simulink model "fwv_modified"  (R2021b)
settings: Solver=ode15s  StartTime=0.0  StopTime=10  FixedStep=0.01  MaxStep=0.01  RelTol=1e-3  AbsTol=1e-3  EnableMultiTasking=on
model workspace (MATLAB code in the model file):
  | p0=[0 0 0];
undefined symbols (not defined in the file): A_D, A_L, adpk, adps, c_bar, C_D0, il, ol, psi0, r00, r11, r22, r33, r_cp, rho, Rw, X, Y, Z, z00, z11, z22, zrd
libraries: sm_lib x54, nesl_utility x45, vrlib x3
(part 3 of 3)

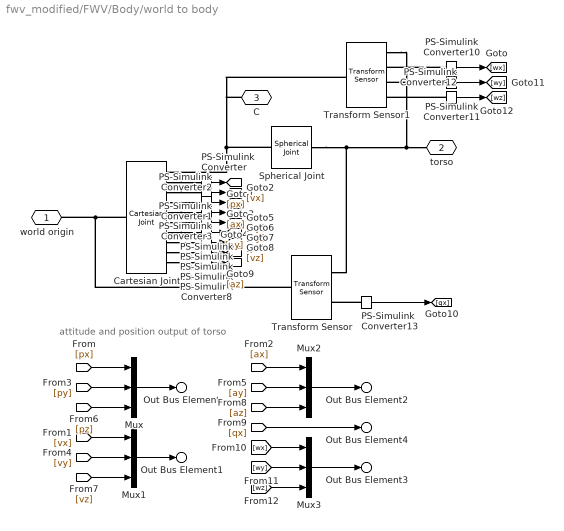
== system fwv_modified/FWV/Body/world to body ==
  note: attitude and position output of torso
  Cartesian Joint : sm_lib/Joints/Cartesian Joint  JointMode=Normal  SenseConstraintForce=off  SenseConstraintForceX=off  SenseConstraintForceY=off  SenseConstraintForceZ=off  SenseConstraintTorque=off  SenseConstraintTorqueX=off  SenseConstraintTorqueY=off  SenseConstraintTorqueZ=off  SenseTotalForce=off  SenseTotalForceX=off  SenseTotalForceY=off  SenseTotalForceZ=off  SenseTotalTorque=off  SenseTotalTorqueX=off  SenseTotalTorqueY=off  SenseTotalTorqueZ=off  CompositeWrenchDir=FollowerOnBase  CompositeWrenchFrame=BaseFrame  PxEquilibriumPosition=0  PxEquilibriumPositionUnits=m  PxSpringStiffness=0  PxSpringStiffnessUnits=N/m  PxDampingCoefficient=0  PxDampingCoefficientUnits=N/(m/s)  PxTorqueActuationMode=NoTorque  PxMotionActuationMode=ComputedMotion  PxSensePosition=on  PxSenseVelocity=on  PxSenseAcceleration=on  PxSenseTorqueForce=off  PxSenseLowerLimitTorqueForce=off  PxSenseUpperLimitTorqueForce=off  PxLowerLimitSpecify=off  PxLowerLimitBound=-1  PxLowerLimitBoundUnits=m  PxLowerLimitStiffness=1e6  PxLowerLimitStiffnessUnits=N/m  PxLowerLimitDamping=1e3  PxLowerLimitDampingUnits=N/(m/s)  PxLowerLimitTransitionRegionWidth=1e-4  PxLowerLimitTransitionRegionWidthUnits=m  PxUpperLimitSpecify=off  PxUpperLimitBound=1  PxUpperLimitBoundUnits=m  PxUpperLimitStiffness=1e6  PxUpperLimitStiffnessUnits=N/m  PxUpperLimitDamping=1e3  PxUpperLimitDampingUnits=N/(m/s)  PxUpperLimitTransitionRegionWidth=1e-4  PxUpperLimitTransitionRegionWidthUnits=m  PxPositionTargetSpecify=on  PxPositionTargetPriority=High  PxPositionTargetValue=p0(1)  PxPositionTargetValueUnits=m  PxVelocityTargetSpecify=off  PxVelocityTargetPriority=High  PxVelocityTargetValue=0  PxVelocityTargetValueUnits=m/s  PyEquilibriumPosition=0  PyEquilibriumPositionUnits=m  PySpringStiffness=0  PySpringStiffnessUnits=N/m  PyDampingCoefficient=0  PyDampingCoefficientUnits=N/(m/s)  PyTorqueActuationMode=NoTorque  PyMotionActuationMode=ComputedMotion  PySensePosition=on  PySenseVelocity=on  PySenseAcceleration=on  PySenseTorqueForce=off  PySenseLowerLimitTorqueForce=off  PySenseUpperLimitTorqueForce=off  PyLowerLimitSpecify=off  PyLowerLimitBound=-1  PyLowerLimitBoundUnits=m  PyLowerLimitStiffness=1e6  PyLowerLimitStiffnessUnits=N/m  PyLowerLimitDamping=1e3  PyLowerLimitDampingUnits=N/(m/s)  PyLowerLimitTransitionRegionWidth=1e-4  PyLowerLimitTransitionRegionWidthUnits=m  PyUpperLimitSpecify=off  PyUpperLimitBound=1  PyUpperLimitBoundUnits=m  PyUpperLimitStiffness=1e6  PyUpperLimitStiffnessUnits=N/m  PyUpperLimitDamping=1e3  PyUpperLimitDampingUnits=N/(m/s)  PyUpperLimitTransitionRegionWidth=1e-4  PyUpperLimitTransitionRegionWidthUnits=m  PyPositionTargetSpecify=on  PyPositionTargetPriority=High  PyPositionTargetValue=p0(2)  PyPositionTargetValueUnits=m  PyVelocityTargetSpecify=off  PyVelocityTargetPriority=High  PyVelocityTargetValue=0  PyVelocityTargetValueUnits=m/s  PzEquilibriumPosition=0  PzEquilibriumPositionUnits=m  PzSpringStiffness=0  PzSpringStiffnessUnits=N/m  PzDampingCoefficient=0  PzDampingCoefficientUnits=N/(m/s)  PzTorqueActuationMode=NoTorque  PzMotionActuationMode=ComputedMotion  PzSensePosition=on  PzSenseVelocity=on  PzSenseAcceleration=on  PzSenseTorqueForce=off  PzSenseLowerLimitTorqueForce=off  PzSenseUpperLimitTorqueForce=off  PzLowerLimitSpecify=off  PzLowerLimitBound=-1  PzLowerLimitBoundUnits=m  PzLowerLimitStiffness=1e6  PzLowerLimitStiffnessUnits=N/m  PzLowerLimitDamping=1e3  PzLowerLimitDampingUnits=N/(m/s)  PzLowerLimitTransitionRegionWidth=1e-4  PzLowerLimitTransitionRegionWidthUnits=m  PzUpperLimitSpecify=off  PzUpperLimitBound=1  PzUpperLimitBoundUnits=m  PzUpperLimitStiffness=1e6  PzUpperLimitStiffnessUnits=N/m  PzUpperLimitDamping=1e3  PzUpperLimitDampingUnits=N/(m/s)  PzUpperLimitTransitionRegionWidth=1e-4  PzUpperLimitTransitionRegionWidthUnits=m  PzPositionTargetSpecify=on  PzPositionTargetPriority=High  PzPositionTargetValue=p0(3)  PzPositionTargetValueUnits=m  PzVelocityTargetSpecify=off  PzVelocityTargetPriority=High  PzVelocityTargetValue=0  PzVelocityTargetValueUnits=m/s
  Mux{,1..3} (4 alike) : Mux  Inputs=3
  PS-Simulink Converter{,1..8,10..13} (13 alike) : nesl_utility/PS-Simulink Converter  PhysicalDomain=network_engine_domain  SubClassName=ps_output  LeftPortType=input  RightPortType=output  PseudoPeriodic=off  Frequencies=[]  Unit=inherit  AffineConversion=off
      settings: SourceProductBaseCode=PW,SS
  Spherical Joint : sm_lib/Joints/Spherical Joint  JointMode=Normal  SenseConstraintForce=off  SenseConstraintForceX=off  SenseConstraintForceY=off  SenseConstraintForceZ=off  SenseConstraintTorque=off  SenseConstraintTorqueX=off  SenseConstraintTorqueY=off  SenseConstraintTorqueZ=off  SenseTotalForce=off  SenseTotalForceX=off  SenseTotalForceY=off  SenseTotalForceZ=off  SenseTotalTorque=off  SenseTotalTorqueX=off  SenseTotalTorqueY=off  SenseTotalTorqueZ=off  CompositeWrenchDir=FollowerOnBase  CompositeWrenchFrame=BaseFrame  DefPosRotationMethod=None  DefPosRotationAngleUnits=deg  DefPosRotationStandardAxis=+Z  DefPosRotationAngle=0.0  DefPosRotationArbitraryAxis=[0 0 1]  DefPosFollAlignAxisA=+X  DefPosBaseAlignAxisA=+Y  DefPosFollAlignAxisB=+Y  DefPosBaseAlignAxisB=+Z  DefPosRotationSequenceAxes=FollowerAxes  DefPosRotationSequence=XYX  DefPosRotationSequenceAngles=[0 0 0]  DefPosRotationSequenceAnglesUnits=deg  DefPosRotationMatrix=[1 0 0; 0 1 0; 0 0 1]  EqPosRotationMethod=None  EqPosRotationAngleUnits=deg  EqPosRotationStandardAxis=+Z  EqPosRotationAngle=0.0  EqPosRotationArbitraryAxis=[0 0 1]  EqPosFollAlignAxisA=+X  EqPosBaseAlignAxisA=+Y  EqPosFollAlignAxisB=+Y  EqPosBaseAlignAxisB=+Z  EqPosRotationSequenceAxes=FollowerAxes  EqPosRotationSequence=XYX  EqPosRotationSequenceAngles=[0 0 0]  EqPosRotationSequenceAnglesUnits=deg  EqPosRotationMatrix=[1 0 0; 0 1 0; 0 0 1]  SpringStiffness=0  SpringStiffnessUnits=N*m/deg  DampingCoefficient=0  DampingCoefficientUnits=N*m/(deg/s)  ActuateTorqueX=off  ActuateTorqueY=off  ActuateTorqueZ=off  ActuateTorque=off  TorqueActuationMode=NoTorque  MotionActuationMode=ComputedMotion  ActuationFrame=BaseFrame  SensePosition=off  SenseVelocityX=off  SenseVelocityY=off  SenseVelocityZ=off  SenseVelocity=off  SenseAccelerationX=off  SenseAccelerationY=off  SenseAccelerationZ=off  SenseAcceleration=off  SenseTorqueX=off  SenseTorqueY=off  SenseTorqueZ=off  SenseTorqueForce=off  SenseLowerLimitTorqueMag=off  SenseUpperLimitTorqueMag=off  SensingFrame=BaseFrame  LowerLimitSpecify=off  LowerLimitBound=15  LowerLimitBoundUnits=deg  LowerLimitStiffness=1e4  LowerLimitStiffnessUnits=N*m/deg  LowerLimitDamping=10  LowerLimitDampingUnits=N*m/(deg/s)  LowerLimitTransitionRegionWidth=0.1  LowerLimitTransitionRegionWidthUnits=deg  UpperLimitSpecify=off  UpperLimitBound=45  UpperLimitBoundUnits=deg  UpperLimitStiffness=1e4  UpperLimitStiffnessUnits=N*m/deg  UpperLimitDamping=10  UpperLimitDampingUnits=N*m/(deg/s)  UpperLimitTransitionRegionWidth=0.1  UpperLimitTransitionRegionWidthUnits=deg  PositionTargetRotationMethod=RotationSequence  PositionTargetRotationAngleUnits=deg  PositionTargetRotationStandardAxis=+Z  PositionTargetRotationAngle=0.0  PositionTargetRotationArbitraryAxis=[0 0 1]  PositionTargetFollAlignAxisA=+X  PositionTargetBaseAlignAxisA=+Y  PositionTargetFollAlignAxisB=+Y  PositionTargetBaseAlignAxisB=+Z  PositionTargetRotationSequenceAxes=FollowerAxes  PositionTargetRotationSequence=ZYX  PositionTargetRotationSequenceAngles=[psi0 theta0 phi0]  PositionTargetRotationSequenceAnglesUnits=rad  PositionTargetRotationMatrix=[1 0 0; 0 1 0; 0 0 1]  PositionTargetSpecify=on  PositionTargetPriority=High  VelocityTargetValue=[0 0 0]  VelocityTargetValueUnits=deg/s  VelocityTargetSpecify=off  VelocityTargetPriority=High  VelocityTargetInFollowerFrame=on
  Transform Sensor : sm_lib/Frames and Transforms/Transform Sensor  MeasurementFrame=NonRotatingBase  SenseAngle=off  SenseAxis=off  SenseAngle1=off  SenseAngle2=off  SenseAngle3=off  SenseQ=off  SenseR=on  SenseOmegaX=off  SenseOmegaY=off  SenseOmegaZ=off  SenseOmega1=off  SenseOmega2=off  SenseOmega3=off  SenseQDot=off  SenseRDot=off  SenseAlphaX=off  SenseAlphaY=off  SenseAlphaZ=off  SenseAlpha1=off  SenseAlpha2=off  SenseAlpha3=off  SenseQDDot=off  SenseRDDot=off  SenseX=off  SenseY=off  SenseZ=off  SenseRad=off  SenseAzim=off  SenseDist=off  SenseInc=off  SenseXDot=off  SenseYDot=off  SenseZDot=off  SenseRadDot=off  SenseAzimDot=off  SenseDistDot=off  SenseIncDot=off  SenseXDDot=off  SenseYDDot=off  SenseZDDot=off  SenseRadDDot=off  SenseAzimDDot=off  SenseDistDDot=off  SenseIncDDot=off
  Transform Sensor1 : sm_lib/Frames and Transforms/Transform Sensor  MeasurementFrame=NonRotatingFollower  SenseAngle=off  SenseAxis=off  SenseAngle1=off  SenseAngle2=off  SenseAngle3=off  SenseQ=off  SenseR=off  SenseOmegaX=on  SenseOmegaY=on  SenseOmegaZ=on  SenseOmega1=off  SenseOmega2=off  SenseOmega3=off  SenseQDot=off  SenseRDot=off  SenseAlphaX=off  SenseAlphaY=off  SenseAlphaZ=off  SenseAlpha1=off  SenseAlpha2=off  SenseAlpha3=off  SenseQDDot=off  SenseRDDot=off  SenseX=off  SenseY=off  SenseZ=off  SenseRad=off  SenseAzim=off  SenseDist=off  SenseInc=off  SenseXDot=off  SenseYDot=off  SenseZDot=off  SenseRadDot=off  SenseAzimDot=off  SenseDistDot=off  SenseIncDot=off  SenseXDDot=off  SenseYDDot=off  SenseZDDot=off  SenseRadDDot=off  SenseAzimDDot=off  SenseDistDDot=off  SenseIncDDot=off
  world origin : PMIOPort  Side=Left
  torso : PMIOPort  Port=2  Side=Right
  C : PMIOPort  Port=3  Side=Left
  Out Bus Element : Outport  PortName=torso_  Element=p
  Out Bus Element1 : Outport  PortName=torso_  Element=v
  Out Bus Element2 : Outport  PortName=torso_  Element=a
  Out Bus Element3 : Outport  PortName=torso_  Element=w
  Out Bus Element4 : Outport  PortName=torso_  Element=R
  wires:
  [vy] -> Mux1/2
  [px] -> Mux/1
  [ax] -> Mux2/1
  [vz] -> Mux1/3
  Mux1/1 -> Out Bus Element1/1
  [az] -> Mux2/3
  [vx] -> Mux1/1
  [ay] -> Mux2/2
  [pz] -> Mux/3
  Mux/1 -> Out Bus Element/1
  Mux2/1 -> Out Bus Element2/1
  [py] -> Mux/2
  PS-Simulink Converter7/1 -> [vz]
  PS-Simulink Converter4/1 -> [vy]
  PS-Simulink Converter5/1 -> [ay]
  PS-Simulink Converter1/1 -> [vx]
  PS-Simulink Converter3/1 -> [py]
  PS-Simulink Converter/1 -> [px]
  PS-Simulink Converter2/1 -> [ax]
  PS-Simulink Converter6/1 -> [pz]
  PS-Simulink Converter8/1 -> [az]
  [qx] -> Out Bus Element4/1
  PS-Simulink Converter13/1 -> [qx]
  PS-Simulink Converter10/1 -> [wx]
  PS-Simulink Converter11/1 -> [wy]
  PS-Simulink Converter12/1 -> [wz]
  Mux3/1 -> Out Bus Element3/1
  [wx] -> Mux3/1
  [wy] -> Mux3/2
  [wz] -> Mux3/3
  connections:
  Cartesian Joint/LConn1 -- world origin/RConn1 -- Transform Sensor/LConn1
  Transform Sensor/RConn1 -- Transform Sensor1/RConn1 -- torso/RConn1 -- Spherical Joint/RConn1
  Spherical Joint/LConn1 -- Transform Sensor1/LConn1 -- C/RConn1 -- Cartesian Joint/RConn1
  PS-Simulink Converter13/LConn1 -- Transform Sensor/RConn2
  Cartesian Joint/RConn2 -- PS-Simulink Converter/LConn1
  Cartesian Joint/RConn3 -- PS-Simulink Converter1/LConn1
  Cartesian Joint/RConn4 -- PS-Simulink Converter2/LConn1
  Cartesian Joint/RConn5 -- PS-Simulink Converter3/LConn1
  Cartesian Joint/RConn6 -- PS-Simulink Converter4/LConn1
  Cartesian Joint/RConn7 -- PS-Simulink Converter5/LConn1
  Cartesian Joint/RConn8 -- PS-Simulink Converter6/LConn1
  Cartesian Joint/RConn9 -- PS-Simulink Converter7/LConn1
  Cartesian Joint/RConn10 -- PS-Simulink Converter8/LConn1
  PS-Simulink Converter10/LConn1 -- Transform Sensor1/RConn2
  PS-Simulink Converter11/LConn1 -- Transform Sensor1/RConn3
  PS-Simulink Converter12/LConn1 -- Transform Sensor1/RConn4

== system fwv_modified/FWV/Controller/Inner PD ==
  eR : Inport
  omega : Inport  Port=2
  Add : Sum  Inputs=---
  Integrator : Integrator  Commented=on  InitialCondition=[0; 0; 0]
  Kd : Constant  Value=diag(il.Kd)
  Kp : Constant  Value=diag(il.Kp)
  Multiply : Gain  Commented=on  Gain=[0.1 0.1 0]
  Product : Product  Multiplication=Matrix(*)
  Product1 : Product  Multiplication=Matrix(*)
  Scope : Scope  NumInputPorts=2
  Selector : Selector  InputPortWidth=3  IndexOptions=Index vector (dialog)  Indices=[2]  OutputSizes=1
  Selector1 : Selector  InputPortWidth=3  IndexOptions=Index vector (dialog)  Indices=[2]  OutputSizes=1
  get P : Subsystem
  to euler1 : Subsystem
  tau_d : Outport
  wires:
  eR/1 -> to euler1/1(R), get P/1(eR)
  Kp/1 -> Product/1
  get P/1(Out) -> Integrator/1, Product/2
  Add/1 -> tau_d/1
  Product1/1 -> Selector1/1, Add/3
  Kd/1 -> Product1/1
  Product/1 -> Selector/1, Add/1
  Selector/1 -> Scope/1
  Selector1/1 -> Scope/2
  omega/1 -> Product1/2
  Integrator/1 -> Multiply/1
  Multiply/1 -> Add/2

== system fwv_modified/FWV/Controller/Mean3 ==
  In1 : Inport
  Add : Sum  Inputs=+-
  Gain : Gain  Gain=1/0.04
  Integrator : Integrator  ZeroCross=off
  Transport Delay : TransportDelay  DelayTime=0.04  InitialOutput=p0  BufferSize=4096
  Mean1 : Outport
  wires:
  In1/1 -> Integrator/1
  Integrator/1 -> Transport Delay/1, Add/1
  Transport Delay/1 -> Add/2
  Add/1 -> Gain/1
  Gain/1 -> Mean1/1

== system fwv_modified/FWV/Controller/Mean4 ==
  In1 : Inport
  Add : Sum  Inputs=+-
  Gain : Gain  Gain=1/0.04
  Integrator : Integrator  ZeroCross=off
  Transport Delay : TransportDelay  DelayTime=0.04  InitialOutput=[0;0;0]  BufferSize=4096
  Mean1 : Outport
  wires:
  In1/1 -> Integrator/1
  Integrator/1 -> Transport Delay/1, Add/1
  Transport Delay/1 -> Add/2
  Add/1 -> Gain/1
  Gain/1 -> Mean1/1

== system fwv_modified/FWV/Controller/Mean5 ==
  In1 : Inport
  Add : Sum  Inputs=+-
  Gain : Gain  Gain=1/0.04
  Integrator : Integrator  ZeroCross=off
  Transport Delay : TransportDelay  DelayTime=0.04  InitialOutput=[0;0;0]  BufferSize=4096
  Mean1 : Outport
  wires:
  In1/1 -> Integrator/1
  Integrator/1 -> Transport Delay/1, Add/1
  Transport Delay/1 -> Add/2
  Add/1 -> Gain/1
  Gain/1 -> Mean1/1

== system fwv_modified/FWV/Controller/Outer PD ==
  ep : Inport
  ev : Inport  Port=2
  a : Inport  Port=3
  Demux : Demux  Outputs=3
  Demux1 : Demux  Outputs=3
  Demux2 : Demux  Outputs=3
  Mux : Mux  Inputs=3
  x PD : Subsystem
  y PD : Subsystem
  z PD : Subsystem
  mu : Outport
  wires:
  ev/1 -> Demux1/1
  a/1 -> Demux2/1
  Demux1/2 -> y PD/2(In2)
  Demux2/3 -> z PD/3(In3)
  Demux2/2 -> y PD/3(In3)
  Demux1/1 -> x PD/2(In2)
  Demux1/3 -> z PD/2(In2)
  Demux/3 -> z PD/1(In1)
  Demux2/1 -> x PD/3(In3)
  Demux/1 -> x PD/1(In1)
  Demux/2 -> y PD/1(In1)
  ep/1 -> Demux/1
  x PD/1(Out1) -> Mux/1
  y PD/1(Out1) -> Mux/2
  z PD/1(Out1) -> Mux/3
  Mux/1 -> mu/1

== system fwv_modified/FWV/Controller/R to euler ==
  R : Inport
  Mux : Mux  Inputs=3
  R to X-Y-Z Extrinsic : Subsystem  mask(Rotation Matrix to X-Y-Z Extrinsic){}
      mask help: Computes roll / pitch / yaw values assuming they correspond to X, Y, and Z rotations, applied in that order and using extrinsic rotations (rotations applied about the fixed axes of the base frame). Does not handle case where Y (pitch) rotation is +/-90 degrees.
  Terminator : Terminator
  rad2deg : Gain  Gain=180/pi
  wires:
  R/1 -> R to X-Y-Z Extrinsic/1(R)
  R to X-Y-Z Extrinsic/2(pitch) -> Mux/2
  Mux/1 -> rad2deg/1
  rad2deg/1 -> Terminator/1
  R to X-Y-Z Extrinsic/1(roll) -> Mux/1
  R to X-Y-Z Extrinsic/3(yaw) -> Mux/3

== system fwv_modified/FWV/Controller/Rd to euler ==
  R : Inport
  R to X-Y-Z Extrinsic : Subsystem  mask(Rotation Matrix to X-Y-Z Extrinsic){}
      mask help: Computes roll / pitch / yaw values assuming they correspond to X, Y, and Z rotations, applied in that order and using extrinsic rotations (rotations applied about the fixed axes of the base frame). Does not handle case where Y (pitch) rotation is +/-90 degrees.
  Terminator : Terminator
  dest euler angles : Mux  Inputs=3
  wires:
  dest euler angles/1 -> Terminator/1
  R/1 -> R to X-Y-Z Extrinsic/1(R)
  R to X-Y-Z Extrinsic/3(yaw) -> dest euler angles/3
  R to X-Y-Z Extrinsic/1(roll) -> dest euler angles/1
  R to X-Y-Z Extrinsic/2(pitch) -> dest euler angles/2

== system fwv_modified/FWV/Controller/adaptive mapping estimator ==
  mu : Inport
  Integrator : Integrator  InitialCondition=0.05
  update k_hat : MATLAB Function  TreatAsAtomicUnit=on
  k_hat : Outport
  wires:
  update k_hat/1(k_hat_dot) -> Integrator/1
  mu/1 -> update k_hat/1(mu)
  Integrator/1 -> update k_hat/2(k_hat), k_hat/1

== system fwv_modified/FWV/Controller/adaptive mapping estimator1 ==
  vd : Inport
  mu : Inport  Port=2
  Abs : Abs  ZeroCross=off
  Integrator : Integrator  InitialCondition=[0; 0; 0]
  MATLAB Function : MATLAB Function  TreatAsAtomicUnit=on
  Product : Product
  Delta_mu : Outport
  wires:
  Product/1 -> Delta_mu/1
  MATLAB Function/1(k_dot) -> Integrator/1
  mu/1 -> MATLAB Function/1(mu)
  Integrator/1 -> Product/2
  vd/1 -> Abs/1, MATLAB Function/2(vd)
  Abs/1 -> Product/1

== system fwv_modified/FWV/Controller/averaged R to euler ==
  R : Inport
  R to X-Y-Z Extrinsic : Subsystem  mask(Rotation Matrix to X-Y-Z Extrinsic){}
      mask help: Computes roll / pitch / yaw values assuming they correspond to X, Y, and Z rotations, applied in that order and using extrinsic rotations (rotations applied about the fixed axes of the base frame). Does not handle case where Y (pitch) rotation is +/-90 degrees.
  Terminator : Terminator
  averaged euler angles : Mux  Inputs=3
  wires:
  R/1 -> R to X-Y-Z Extrinsic/1(R)
  R to X-Y-Z Extrinsic/2(pitch) -> averaged euler angles/2
  averaged euler angles/1 -> Terminator/1
  R to X-Y-Z Extrinsic/1(roll) -> averaged euler angles/1
  R to X-Y-Z Extrinsic/3(yaw) -> averaged euler angles/3

== system fwv_modified/FWV/Controller/period averaging ==
  in : Inport
  MATLAB Function : MATLAB Function  TreatAsAtomicUnit=on
  Mean : Subsystem
  Mean1 : Outport
  wires:
  in/1 -> Mean/1(In1)
  Mean/1(Out1) -> MATLAB Function/1(R_raw)
  MATLAB Function/1(R_mean) -> Mean1/1

== system fwv_modified/FWV/Visualization/Subsystem ==
  R : Inport
  Atan1 : Trigonometry  Operator=atan2
  Demux1 : Demux  Outputs=2
  "R([2 1], 1)" : Selector  NumberOfDimensions=2  InputPortWidth=3  IndexOptions=Index vector (dialog),Index vector (dialog)  Indices=[2 1],1  OutputSizes=1,1
  Reshape : Reshape
  yaw : Outport  VectorParamsAs1DForOutWhenUnconnected=off
  wires:
  "R([2 1], 1)"/1 -> Demux1/1
  Atan1/1 -> Reshape/1
  Demux1/1 -> Atan1/1
  Reshape/1 -> yaw/1
  Demux1/2 -> Atan1/2
  R/1 -> "R([2 1], 1)"/1

== system fwv_modified/FWV/Body/LEFT WING/Subsystem1 ==
  Gain : Gain  Gain=-1
  LWing-root in world : sm_lib/Frames and Transforms/Transform Sensor  MeasurementFrame=NonRotatingFollower  SenseAngle=off  SenseAxis=off  SenseAngle1=off  SenseAngle2=off  SenseAngle3=off  SenseQ=off  SenseR=off  SenseOmegaX=on  SenseOmegaY=on  SenseOmegaZ=off  SenseOmega1=off  SenseOmega2=off  SenseOmega3=off  SenseQDot=off  SenseRDot=off  SenseAlphaX=off  SenseAlphaY=off  SenseAlphaZ=off  SenseAlpha1=off  SenseAlpha2=off  SenseAlpha3=off  SenseQDDot=off  SenseRDDot=off  SenseX=off  SenseY=off  SenseZ=off  SenseRad=off  SenseAzim=off  SenseDist=off  SenseInc=off  SenseXDot=on  SenseYDot=on  SenseZDot=off  SenseRadDot=off  SenseAzimDot=off  SenseDistDot=off  SenseIncDot=off  SenseXDDot=off  SenseYDDot=off  SenseZDDot=off  SenseRadDDot=off  SenseAzimDDot=off  SenseDistDDot=off  SenseIncDDot=off
  Mux : Mux
  PS-Simulink Converter{,1..3} (4 alike) : nesl_utility/PS-Simulink Converter  PhysicalDomain=network_engine_domain  SubClassName=ps_output  LeftPortType=input  RightPortType=output  PseudoPeriodic=off  Frequencies=[]  Unit=inherit  AffineConversion=off
      settings: SourceProductBaseCode=PW,SS
  W : PMIOPort  Side=Left
  WT : PMIOPort  Port=2  Side=Left
  le0 : Outport
  wires:
  Mux/1 -> le0/1
  Gain/1 -> Mux/2
  PS-Simulink Converter1/1 -> Mux/3
  PS-Simulink Converter3/1 -> Gain/1
  PS-Simulink Converter2/1 -> Mux/1
  PS-Simulink Converter/1 -> Mux/4
  connections:
  W/RConn1 -- LWing-root in world/LConn1
  WT/RConn1 -- LWing-root in world/RConn1
  LWing-root in world/RConn2 -- PS-Simulink Converter/LConn1
  LWing-root in world/RConn3 -- PS-Simulink Converter1/LConn1
  LWing-root in world/RConn4 -- PS-Simulink Converter2/LConn1
  LWing-root in world/RConn5 -- PS-Simulink Converter3/LConn1

== system fwv_modified/FWV/Body/RIGHT WING/Subsystem1 ==
  Gain : Gain  Gain=-1
  LWing-root in world : sm_lib/Frames and Transforms/Transform Sensor  MeasurementFrame=NonRotatingFollower  SenseAngle=off  SenseAxis=off  SenseAngle1=off  SenseAngle2=off  SenseAngle3=off  SenseQ=off  SenseR=off  SenseOmegaX=on  SenseOmegaY=on  SenseOmegaZ=off  SenseOmega1=off  SenseOmega2=off  SenseOmega3=off  SenseQDot=off  SenseRDot=off  SenseAlphaX=off  SenseAlphaY=off  SenseAlphaZ=off  SenseAlpha1=off  SenseAlpha2=off  SenseAlpha3=off  SenseQDDot=off  SenseRDDot=off  SenseX=off  SenseY=off  SenseZ=off  SenseRad=off  SenseAzim=off  SenseDist=off  SenseInc=off  SenseXDot=on  SenseYDot=on  SenseZDot=off  SenseRadDot=off  SenseAzimDot=off  SenseDistDot=off  SenseIncDot=off  SenseXDDot=off  SenseYDDot=off  SenseZDDot=off  SenseRadDDot=off  SenseAzimDDot=off  SenseDistDDot=off  SenseIncDDot=off
  Mux : Mux
  PS-Simulink Converter{,1..3} (4 alike) : nesl_utility/PS-Simulink Converter  PhysicalDomain=network_engine_domain  SubClassName=ps_output  LeftPortType=input  RightPortType=output  PseudoPeriodic=off  Frequencies=[]  Unit=inherit  AffineConversion=off
      settings: SourceProductBaseCode=PW,SS
  W : PMIOPort  Side=Left
  WT : PMIOPort  Port=2  Side=Left
  le0 : Outport
  wires:
  Mux/1 -> le0/1
  Gain/1 -> Mux/2
  PS-Simulink Converter1/1 -> Mux/3
  PS-Simulink Converter3/1 -> Gain/1
  PS-Simulink Converter2/1 -> Mux/1
  PS-Simulink Converter/1 -> Mux/4
  connections:
  W/RConn1 -- LWing-root in world/LConn1
  WT/RConn1 -- LWing-root in world/RConn1
  LWing-root in world/RConn2 -- PS-Simulink Converter/LConn1
  LWing-root in world/RConn3 -- PS-Simulink Converter1/LConn1
  LWing-root in world/RConn4 -- PS-Simulink Converter2/LConn1
  LWing-root in world/RConn5 -- PS-Simulink Converter3/LConn1

== system fwv_modified/FWV/Controller/Inner PD/get P ==
  eR : Inport
  Add : Sum  Inputs=+++
  Cross Product : vrlib/Utilities/Cross Product
  Cross Product1 : vrlib/Utilities/Cross Product
  Cross Product2 : vrlib/Utilities/Cross Product
  One : Constant  Value=[1;0;0]  OutDataTypeStr=Inherit: Inherit via back propagation
  One1 : Constant  Value=[0;1;0]  OutDataTypeStr=Inherit: Inherit via back propagation
  One2 : Constant  Value=[0;0;1]  OutDataTypeStr=Inherit: Inherit via back propagation
  Product : Product  Multiplication=Matrix(*)
  Product1 : Product  Multiplication=Matrix(*)
  Product2 : Product  Multiplication=Matrix(*)
  Out : Outport
  wires:
  One/1 -> Product/2, Cross Product/1
  One1/1 -> Cross Product1/1, Product1/2
  One2/1 -> Cross Product2/1, Product2/2
  eR/1 -> Product/1, Product1/1, Product2/1
  Cross Product/1 -> Add/1
  Cross Product1/1 -> Add/2
  Cross Product2/1 -> Add/3
  Add/1 -> Out/1
  Product/1 -> Cross Product/2
  Product1/1 -> Cross Product1/2
  Product2/1 -> Cross Product2/2

== system fwv_modified/FWV/Controller/Inner PD/to euler1 ==
  R : Inport
  R to X-Y-Z Extrinsic : Subsystem  mask(Rotation Matrix to X-Y-Z Extrinsic){}
      mask help: Computes roll / pitch / yaw values assuming they correspond to X, Y, and Z rotations, applied in that order and using extrinsic rotations (rotations applied about the fixed axes of the base frame). Does not handle case where Y (pitch) rotation is +/-90 degrees.
  Terminator : Terminator
  euler angle differences : Mux  Inputs=3
  wires:
  euler angle differences/1 -> Terminator/1
  R/1 -> R to X-Y-Z Extrinsic/1(R)
  R to X-Y-Z Extrinsic/3(yaw) -> euler angle differences/3
  R to X-Y-Z Extrinsic/1(roll) -> euler angle differences/1
  R to X-Y-Z Extrinsic/2(pitch) -> euler angle differences/2

== system fwv_modified/FWV/Controller/Outer PD/x PD ==
  In1 : Inport
  In2 : Inport  Port=2
  In3 : Inport  Port=3
  Add : Sum  Inputs=++++
  Constant : Constant  Value=ol.Kp(1)
  Constant1 : Constant  Value=0
  Constant2 : Constant  Value=ol.Kd(1)
  Gain : Gain
  Integrator Limited : Integrator  UpperSaturationLimit=1  LowerSaturationLimit=0
  Product : Product
  Product1 : Product
  Product2 : Product
  Scope : Scope  NumInputPorts=2
  Out1 : Outport
  wires:
  Add/1 -> Out1/1
  In1/1 -> Product1/2, Product/2
  Product/1 -> Scope/1, Add/1
  Constant/1 -> Product/1
  Product2/1 -> Scope/2, Add/3
  In2/1 -> Product2/2
  Constant2/1 -> Product2/1
  Integrator Limited/1 -> Add/2
  Product1/1 -> Integrator Limited/1
  Constant1/1 -> Product1/1
  In3/1 -> Gain/1
  Gain/1 -> Add/4

== system fwv_modified/FWV/Controller/Outer PD/y PD ==
  In1 : Inport
  In2 : Inport  Port=2
  In3 : Inport  Port=3
  Add : Sum  Inputs=++++
  Constant : Constant  Value=ol.Kp(2)
  Constant1 : Constant  Value=0
  Constant2 : Constant  Value=ol.Kd(2)
  Gain : Gain
  Integrator Limited : Integrator  UpperSaturationLimit=1  LowerSaturationLimit=0
  Product : Product
  Product1 : Product
  Product2 : Product
  Out1 : Outport
  wires:
  Add/1 -> Out1/1
  In1/1 -> Product1/2, Product/2
  Product/1 -> Add/1
  Constant/1 -> Product/1
  Product2/1 -> Add/3
  In2/1 -> Product2/2
  Constant2/1 -> Product2/1
  Integrator Limited/1 -> Add/2
  Product1/1 -> Integrator Limited/1
  Constant1/1 -> Product1/1
  In3/1 -> Gain/1
  Gain/1 -> Add/4

== system fwv_modified/FWV/Controller/Outer PD/z PD ==
  In1 : Inport
  In2 : Inport  Port=2
  In3 : Inport  Port=3
  Add : Sum  Inputs=++++
  Constant : Constant  Value=ol.Kp(3)
  Constant1 : Constant  Value=0
  Constant2 : Constant  Value=ol.Kd(3)
  Integrator Limited : Integrator  UpperSaturationLimit=5  LowerSaturationLimit=-5
  Product : Product
  Product1 : Product
  Product2 : Product
  Scope : Scope
  Scope1 : Scope
  Out1 : Outport
  wires:
  Add/1 -> Out1/1
  In1/1 -> Product1/2, Scope/1, Product/2
  Product/1 -> Add/1
  Constant/1 -> Product/1
  Product2/1 -> Add/3
  In2/1 -> Scope1/1, Product2/2
  Constant2/1 -> Product2/1
  Integrator Limited/1 -> Add/2
  Product1/1 -> Integrator Limited/1
  Constant1/1 -> Product1/1
  In3/1 -> Add/4

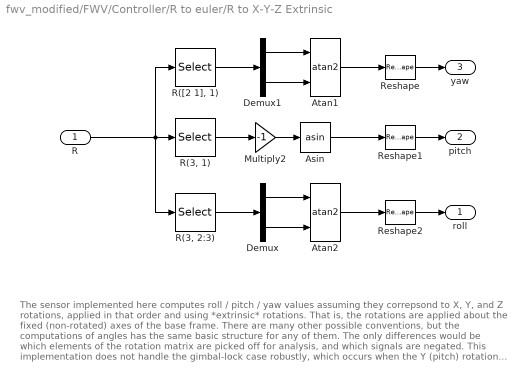
== system fwv_modified/FWV/Controller/R to euler/R to X-Y-Z Extrinsic ==
  note: The sensor implemented here computes roll / pitch / yaw values assuming they correpsond to X, Y, and Z rotations, applied in that order and using  *extrinsic* rotations.  That is, the rotations are applied about the fixed (non-rotated) axes of the base frame.   There are many other possible conventions, but the computations of angles has the same basic structure for any of them.  The only differences would be which elements of the rotation matrix are picked off for analysis, and which signals are negated.
      |
      | This implementation does not handle the gimbal-lock case robustly, which occurs when the Y (pitch) rotation is +/-90 degrees.  Handling this case requires a more complex computation,
      | but it can be done with a few more trig blocks and selectors.
  R : Inport
  Asin : Trigonometry  Operator=asin
  Atan1 : Trigonometry  Operator=atan2
  Atan2 : Trigonometry  Operator=atan2
  Demux : Demux  Outputs=2
  Demux1 : Demux  Outputs=2
  Multiply2 : Gain  Gain=-1
  "R(3, 1)" : Selector  NumberOfDimensions=2  InputPortWidth=3  IndexOptions=Index vector (dialog),Index vector (dialog)  Indices=3,1  OutputSizes=1,1
  "R(3, 2:3)" : Selector  NumberOfDimensions=2  InputPortWidth=3  IndexOptions=Index vector (dialog),Index vector (dialog)  Indices=3,[2 3]  OutputSizes=1,1
  "R([2 1], 1)" : Selector  NumberOfDimensions=2  InputPortWidth=3  IndexOptions=Index vector (dialog),Index vector (dialog)  Indices=[2 1],1  OutputSizes=1,1
  Reshape : Reshape
  Reshape1 : Reshape
  Reshape2 : Reshape  OutputDimensionality=Customize  OutputDimensions=1
  roll : Outport  VectorParamsAs1DForOutWhenUnconnected=off
  pitch : Outport  Port=2  VectorParamsAs1DForOutWhenUnconnected=off
  yaw : Outport  Port=3  VectorParamsAs1DForOutWhenUnconnected=off
  wires:
  Demux/1 -> Atan2/1
  Demux1/2 -> Atan1/2
  Demux/2 -> Atan2/2
  Atan2/1 -> Reshape2/1
  "R(3, 1)"/1 -> Multiply2/1
  Asin/1 -> Reshape1/1
  R/1 -> "R(3, 1)"/1, "R(3, 2:3)"/1, "R([2 1], 1)"/1
  Demux1/1 -> Atan1/1
  "R([2 1], 1)"/1 -> Demux1/1
  Multiply2/1 -> Asin/1
  "R(3, 2:3)"/1 -> Demux/1
  Atan1/1 -> Reshape/1
  Reshape/1 -> yaw/1
  Reshape1/1 -> pitch/1
  Reshape2/1 -> roll/1

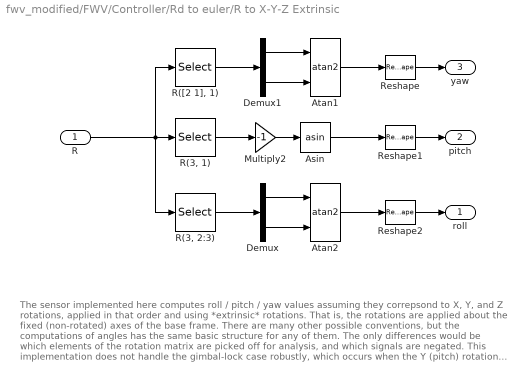
== system fwv_modified/FWV/Controller/Rd to euler/R to X-Y-Z Extrinsic ==
  note: The sensor implemented here computes roll / pitch / yaw values assuming they correpsond to X, Y, and Z rotations, applied in that order and using  *extrinsic* rotations.  That is, the rotations are applied about the fixed (non-rotated) axes of the base frame.   There are many other possible conventions, but the computations of angles has the same basic structure for any of them.  The only differences would be which elements of the rotation matrix are picked off for analysis, and which signals are negated.
      |
      | This implementation does not handle the gimbal-lock case robustly, which occurs when the Y (pitch) rotation is +/-90 degrees.  Handling this case requires a more complex computation,
      | but it can be done with a few more trig blocks and selectors.
  R : Inport
  Asin : Trigonometry  Operator=asin
  Atan1 : Trigonometry  Operator=atan2
  Atan2 : Trigonometry  Operator=atan2
  Demux : Demux  Outputs=2
  Demux1 : Demux  Outputs=2
  Multiply2 : Gain  Gain=-1
  "R(3, 1)" : Selector  NumberOfDimensions=2  InputPortWidth=3  IndexOptions=Index vector (dialog),Index vector (dialog)  Indices=3,1  OutputSizes=1,1
  "R(3, 2:3)" : Selector  NumberOfDimensions=2  InputPortWidth=3  IndexOptions=Index vector (dialog),Index vector (dialog)  Indices=3,[2 3]  OutputSizes=1,1
  "R([2 1], 1)" : Selector  NumberOfDimensions=2  InputPortWidth=3  IndexOptions=Index vector (dialog),Index vector (dialog)  Indices=[2 1],1  OutputSizes=1,1
  Reshape : Reshape
  Reshape1 : Reshape
  Reshape2 : Reshape  OutputDimensionality=Customize  OutputDimensions=1
  roll : Outport  VectorParamsAs1DForOutWhenUnconnected=off
  pitch : Outport  Port=2  VectorParamsAs1DForOutWhenUnconnected=off
  yaw : Outport  Port=3  VectorParamsAs1DForOutWhenUnconnected=off
  wires:
  Demux/1 -> Atan2/1
  Demux1/2 -> Atan1/2
  Demux/2 -> Atan2/2
  Atan2/1 -> Reshape2/1
  "R(3, 1)"/1 -> Multiply2/1
  Asin/1 -> Reshape1/1
  R/1 -> "R(3, 1)"/1, "R(3, 2:3)"/1, "R([2 1], 1)"/1
  Demux1/1 -> Atan1/1
  "R([2 1], 1)"/1 -> Demux1/1
  Multiply2/1 -> Asin/1
  "R(3, 2:3)"/1 -> Demux/1
  Atan1/1 -> Reshape/1
  Reshape/1 -> yaw/1
  Reshape1/1 -> pitch/1
  Reshape2/1 -> roll/1

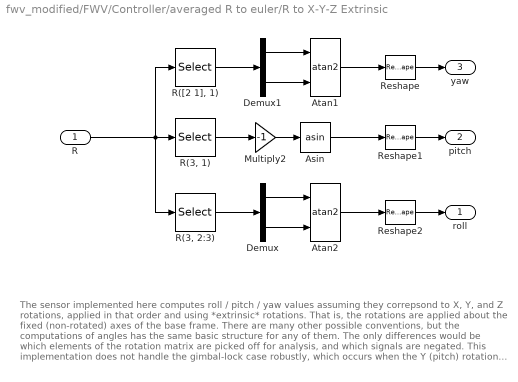
== system fwv_modified/FWV/Controller/averaged R to euler/R to X-Y-Z Extrinsic ==
  note: The sensor implemented here computes roll / pitch / yaw values assuming they correpsond to X, Y, and Z rotations, applied in that order and using  *extrinsic* rotations.  That is, the rotations are applied about the fixed (non-rotated) axes of the base frame.   There are many other possible conventions, but the computations of angles has the same basic structure for any of them.  The only differences would be which elements of the rotation matrix are picked off for analysis, and which signals are negated.
      |
      | This implementation does not handle the gimbal-lock case robustly, which occurs when the Y (pitch) rotation is +/-90 degrees.  Handling this case requires a more complex computation,
      | but it can be done with a few more trig blocks and selectors.
  R : Inport
  Asin : Trigonometry  Operator=asin
  Atan1 : Trigonometry  Operator=atan2
  Atan2 : Trigonometry  Operator=atan2
  Demux : Demux  Outputs=2
  Demux1 : Demux  Outputs=2
  Multiply2 : Gain  Gain=-1
  "R(3, 1)" : Selector  NumberOfDimensions=2  InputPortWidth=3  IndexOptions=Index vector (dialog),Index vector (dialog)  Indices=3,1  OutputSizes=1,1
  "R(3, 2:3)" : Selector  NumberOfDimensions=2  InputPortWidth=3  IndexOptions=Index vector (dialog),Index vector (dialog)  Indices=3,[2 3]  OutputSizes=1,1
  "R([2 1], 1)" : Selector  NumberOfDimensions=2  InputPortWidth=3  IndexOptions=Index vector (dialog),Index vector (dialog)  Indices=[2 1],1  OutputSizes=1,1
  Reshape : Reshape
  Reshape1 : Reshape
  Reshape2 : Reshape  OutputDimensionality=Customize  OutputDimensions=1
  roll : Outport  VectorParamsAs1DForOutWhenUnconnected=off
  pitch : Outport  Port=2  VectorParamsAs1DForOutWhenUnconnected=off
  yaw : Outport  Port=3  VectorParamsAs1DForOutWhenUnconnected=off
  wires:
  Demux/1 -> Atan2/1
  Demux1/2 -> Atan1/2
  Demux/2 -> Atan2/2
  Atan2/1 -> Reshape2/1
  "R(3, 1)"/1 -> Multiply2/1
  Asin/1 -> Reshape1/1
  R/1 -> "R(3, 1)"/1, "R(3, 2:3)"/1, "R([2 1], 1)"/1
  Demux1/1 -> Atan1/1
  "R([2 1], 1)"/1 -> Demux1/1
  Multiply2/1 -> Asin/1
  "R(3, 2:3)"/1 -> Demux/1
  Atan1/1 -> Reshape/1
  Reshape/1 -> yaw/1
  Reshape1/1 -> pitch/1
  Reshape2/1 -> roll/1

== system fwv_modified/FWV/Controller/period averaging/Mean ==
  In1 : Inport
  Add : Sum  Inputs=+-
  Gain : Gain  Gain=1/0.04
  Integrator : Integrator  ZeroCross=off
  Transport Delay : TransportDelay  DelayTime=0.04  InitialOutput=[cos(psi0),-sin(psi0),0;sin(psi0),cos(psi0),0;0,0,1]  BufferSize=4096
  Out1 : Outport
  wires:
  In1/1 -> Integrator/1
  Integrator/1 -> Transport Delay/1, Add/1
  Add/1 -> Gain/1
  Gain/1 -> Out1/1
  Transport Delay/1 -> Add/2

== system fwv_modified/FWV/Controller/Inner PD/to euler1/R to X-Y-Z Extrinsic ==
  note: The sensor implemented here computes roll / pitch / yaw values assuming they correpsond to X, Y, and Z rotations, applied in that order and using  *extrinsic* rotations.  That is, the rotations are applied about the fixed (non-rotated) axes of the base frame.   There are many other possible conventions, but the computations of angles has the same basic structure for any of them.  The only differences would be which elements of the rotation matrix are picked off for analysis, and which signals are negated.
      |
      | This implementation does not handle the gimbal-lock case robustly, which occurs when the Y (pitch) rotation is +/-90 degrees.  Handling this case requires a more complex computation,
      | but it can be done with a few more trig blocks and selectors.
  R : Inport
  Asin : Trigonometry  Operator=asin
  Atan1 : Trigonometry  Operator=atan2
  Atan2 : Trigonometry  Operator=atan2
  Demux : Demux  Outputs=2
  Demux1 : Demux  Outputs=2
  Multiply2 : Gain  Gain=-1
  "R(3, 1)" : Selector  NumberOfDimensions=2  InputPortWidth=3  IndexOptions=Index vector (dialog),Index vector (dialog)  Indices=3,1  OutputSizes=1,1
  "R(3, 2:3)" : Selector  NumberOfDimensions=2  InputPortWidth=3  IndexOptions=Index vector (dialog),Index vector (dialog)  Indices=3,[2 3]  OutputSizes=1,1
  "R([2 1], 1)" : Selector  NumberOfDimensions=2  InputPortWidth=3  IndexOptions=Index vector (dialog),Index vector (dialog)  Indices=[2 1],1  OutputSizes=1,1
  Reshape : Reshape
  Reshape1 : Reshape
  Reshape2 : Reshape  OutputDimensionality=Customize  OutputDimensions=1
  roll : Outport  VectorParamsAs1DForOutWhenUnconnected=off
  pitch : Outport  Port=2  VectorParamsAs1DForOutWhenUnconnected=off
  yaw : Outport  Port=3  VectorParamsAs1DForOutWhenUnconnected=off
  wires:
  Demux/1 -> Atan2/1
  Demux1/2 -> Atan1/2
  Demux/2 -> Atan2/2
  Atan2/1 -> Reshape2/1
  "R(3, 1)"/1 -> Multiply2/1
  Asin/1 -> Reshape1/1
  R/1 -> "R(3, 1)"/1, "R(3, 2:3)"/1, "R([2 1], 1)"/1
  Demux1/1 -> Atan1/1
  "R([2 1], 1)"/1 -> Demux1/1
  Multiply2/1 -> Asin/1
  "R(3, 2:3)"/1 -> Demux/1
  Atan1/1 -> Reshape/1
  Reshape/1 -> yaw/1
  Reshape1/1 -> pitch/1
  Reshape2/1 -> roll/1

== matlab function fwv_modified/FWV/Body/LEFT WING/AoA ==
  data: le0 input; alpha output; rot input; Rw parameter; r33 parameter; r22 parameter
function alpha = fcn(le0, rot, Rw, r33, r22)
rcp = Rw*r33/r22;
vi = le0(1)+le0(3)*rcp;
vo = le0(2)+le0(4)*rcp;
dir_v = atan2(vo,vi);
if vi~=0
    alpha = -rot + sign(vi)*pi/2 - atan(vo/vi);
else
    alpha = 0;
end

== matlab function fwv_modified/FWV/Body/LEFT WING/left aero force and moment ==
  data: le0 input; F_N output; alpha input; M_rd output; M_ae output; d_cp output; rot_dot input; A_L parameter; A_D parameter; C_D0 parameter; rho parameter; c_bar parameter; Rw parameter; r22 parameter; r11 parameter; r00 parameter; z22 parameter; z11 parameter; z00 parameter; zrd parameter
function [F_N, M_rd, M_ae, d_cp] = fcn(le0, alpha, rot_dot, A_L, A_D, C_D0, rho, c_bar, Rw, r22, r11, r00, z22, z11, z00, zrd)
a2=le0(3)^2+le0(4)^2;
a1=2*(le0(1)*le0(3)+le0(2)*le0(4));
a0=le0(1)^2+le0(2)^2;
C_L=A_L*sin(2*alpha);
C_D=C_D0+A_D*(1-cos(2*alpha));
C_N=C_L*cos(alpha)+C_D*sin(alpha);
C_A=C_L*sin(alpha)-C_D*cos(alpha);
F_N = -0.5*rho*C_N*c_bar*(a2*Rw^3*r22+a1*Rw^2*r11+a0*Rw*r00);
d_cp_=0.82/pi*(mod(abs(alpha),pi))+0.05;
M_ae=0.5*rho*C_N*c_bar^2*d_cp_*(a2*Rw^3*z22+a1*Rw^2*z11+a0*Rw*z00);
if F_N==0
    d_cp=-0.51*c_bar;
else
    d_cp = M_ae/F_N;
end
M_rd=-0.125*rho*5*rot_dot*abs(rot_dot)*Rw*c_bar^4*zrd;

== matlab function fwv_modified/FWV/Body/RIGHT WING/AoA1 ==
  data: le0 input; alpha output; rot input; Rw parameter; r33 parameter; r22 parameter
function alpha = fcn(le0, rot, Rw, r33, r22)
rcp = -Rw*r33/r22;
vi = le0(1)+le0(3)*rcp;
vo = le0(2)+le0(4)*rcp;
if vi~=0
    alpha = -rot + sign(vi)*pi/2 - atan(vo/vi);
else
    alpha = 0;
end

== matlab function fwv_modified/FWV/Body/RIGHT WING/right aero force and moment ==
  data: le0 input; F_N output; alpha input; M_rd output; d_cp output; rot_dot input; A_L parameter; A_D parameter; C_D0 parameter; rho parameter; c_bar parameter; Rw parameter; r22 parameter; r11 parameter; r00 parameter; z22 parameter; z11 parameter; z00 parameter; zrd parameter
function [F_N,M_rd,d_cp]= fcn(le0, alpha, rot_dot, A_L, A_D, C_D0, rho, c_bar, Rw, r22, r11, r00, z22, z11, z00, zrd)
a2=le0(3)^2+le0(4)^2;
a1=-2*(le0(1)*le0(3)+le0(2)*le0(4));
a0=le0(1)^2+le0(2)^2;
C_L=A_L*sin(2*alpha);
C_D=C_D0+A_D*(1-cos(2*alpha));
C_N=C_L*cos(alpha)+C_D*sin(alpha);
C_A=C_L*sin(alpha)-C_D*cos(alpha);
F_N = -0.5*rho*C_N*c_bar*(a2*Rw^3*r22+a1*Rw^2*r11+a0*Rw*r00);
d_cp_=0.82/pi*(mod(abs(alpha),pi))+0.05;
M_ae=0.5*rho*C_N*c_bar^2*d_cp_*(a2*Rw^3*z22+a1*Rw^2*z11+a0*Rw*z00);
if F_N==0
    d_cp=-0.51*c_bar;
else
    d_cp=M_ae/F_N;
end
M_rd=-0.125*rho*5*rot_dot*abs(rot_dot)*Rw*c_bar^4*zrd;

== matlab function fwv_modified/Ref/p,pdot,pddot ==
  data: t input; p output; heading output; v output; heading_dot output; a output; heading_ddot output
function [p,heading,v,heading_dot,a,heading_ddot] = fcn(t)
% stablization
p=[0.5; 0.4; 0.8];
heading = pi/3;
heading_dot = 0;
heading_ddot = 0;
v=[0; 0; 0];
a=[0; 0; 0];

% forward flight
% p=[0.5*t; -0.5*t; 0.8];
% heading = -pi/4;
% heading_dot = 0;
% heading_ddot = 0;
% v=[0.5; -0.5; 0];
% a=[0; 0; 0];

% cruising flight
% amp=1;
% omega=pi/3;
% hgt=1;
% p(1)=amp*sin(omega*t);
% p(2)=-amp*cos(omega*t)+amp;
% p(3)=hgt;
% v(1)=amp*omega*cos(omega*t);
% v(2)=amp*omega*sin(omega*t);
% v(3)=0;
% a(1)=-amp*omega*omega*sin(omega*t);
% a(2)=amp*omega*omega*cos(omega*t);
% a(3)=0;
% heading = (omega*t);
% heading = mod(heading + pi, 2*pi)-pi;
% heading_dot = omega;
% heading_ddot = 0;

== matlab function fwv_modified/FWV/Controller/MATLAB Function ==
  data: Rd output size=[3 3]; mu input; k_hat input; amp output; heading input
function [Rd, amp]= fcn(mu, k_hat,heading)
% k_hat=0.05;
amp=k_hat*(mu(3)+9.806);
if amp > 1
    amp = 1;
end
if amp < 0
    amp = 0;
end
Rz=[cos(heading) -sin(heading) 0;
        sin(heading) cos(heading) 0;
        0 0 1];
% mu=Rz*mu;
mu(3)=9.806;
std_mu=mu./norm(mu);

if norm(std_mu-[0;0;1])<1e-2
    Rd=Rz;
else
%     w=cross([0;0;1],std_mu);
%     w=w./norm(w);
%     theta=acos(dot([0;0;1],std_mu));
%     Rd=axang2rotm([w',theta]);
    g1=std_mu(1);g2=std_mu(2);g3=std_mu(3);
    g23=sqrt(g2^2 + g3^2);
    Rd=[g23 0 g1;
        -g1*g2/g23 g3/g23 g2;
        -g1*g3/g23 -g2/g23 g3];
    Rd=Rd*Rz;
end

== matlab function fwv_modified/FWV/Body/TAIL/get F ==
  data: w input; F output
function F = fcn(w)
l_til=0.01;
A_til=3e-4;
F=-0.5*sign(w)*(0.25*l_til*w)^2*A_til;

== matlab function fwv_modified/FWV/Controller/period averaging/MATLAB Function ==
  data: R_raw input; R_mean output
function R_mean = fcn(R_raw)
[U,~,V]=svd(R_raw);
R_mean=U*V';

== matlab function fwv_modified/FWV/Controller/adaptive mapping estimator/update k_hat ==
  data: mu input; k_hat input; k_hat_dot output
function k_hat_dot = fcn(mu,k_hat)
k_hat_dot = 0.005*sign(mu(3))*abs(mu(3))^(1/3);

== matlab function fwv_modified/FWV/Controller/adaptive mapping estimator1/MATLAB Function ==
  data: mu input; k_dot output; vd input; adpk parameter; adps parameter
function k_dot = fcn(mu, vd, adpk, adps)

k_dot = (adpk)*mu./(norm(mu)+adps).*double(abs(vd)-2e-2>0);

== matlab function fwv_modified/FWV/Body/Acuator/ left flap ==
  data: t input; y output; amp input; sig input; freq input; bias input
function y = flap(t,amp,sig,freq,bias)
sig=1-sig;
tn = mod(freq*t,1);
if tn<sig
    y = amp*(cos(2*pi*tn/(2*sig)))+bias;
else
    y = amp*(cos(2*pi*(1-tn)/(2-2*sig)))+bias;
end
if abs(y)>pi/2
    y = sign(y)*pi/2;
end

== matlab function fwv_modified/FWV/Body/Acuator/ right flap ==
  data: t input; y output; amp input; sig input; freq input; bias input
function y = flap(t,amp,sig,freq,bias)
% sig=1-sig;
tn = mod(freq*t,1);
if tn<sig
    y = amp*(cos(2*pi*tn/(2*sig)))+bias;
else
    y = amp*(cos(2*pi*(1-tn)/(2-2*sig)))+bias;
end
if abs(y)>pi/2
    y = sign(y)*pi/2;
end
